simulink model "reverbatinDelay"  (Simulink 7.7)
settings: Solver=FixedStepDiscrete  StartTime=0.0  StopTime=10.0  RelTol=1e-3
libraries: dspsigops x1, dspsrcs4 x1, dspmtrx3 x1, dspsnks4 x1
settings Model: Creator=Arun  LastModifiedBy=Arun

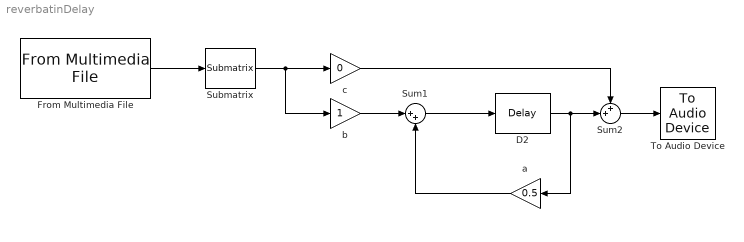
== system reverbatinDelay ==
  D2 : dspsigops/Delay  InputProcessing=Columns as channels (frame based)  dly_unit=Samples  delay=6000  ic_detail=off  dif_ic_for_ch=off  dif_ic_for_dly=off  ic=0  reset_popup=None
  From Multimedia File : dspsrcs4/From Multimedia File  inputFilename=I:\Documents and Settings\Arun\Desktop\monayi\speech_dft.wav  loop=on  numPlays=1  outputStreams=Audio only  videoDataType=single  audioDataType=double  inheritSampleTime=on  userDefinedSampleTime=1/30  noAudioOutput=off  isIntensityVideo=off  fourcc=RGB  colorVideoFormat=Separate color signals  outputEOF=off  dataOrg=Column-major  audioFrameSize=1  computeAudioFrameSize=off
  Submatrix : dspmtrx3/Submatrix  RowSpan=All rows  RowStartMode=First  RowStartIndex=1  RowEndMode=Last  RowEndIndex=1  ColSpan=One column  ColStartMode=First  ColStartIndex=1  ColEndMode=Last  ColEndIndex=1
  Sum1 : Sum  Inputs=|++
  Sum2 : Sum  Inputs=++|
  To Audio Device : dspsnks4/To Audio Device  deviceName=Default  inheritSampleRate=on  sampleRate=44100  deviceDatatype=Determine from input data type  autoBufferSize=on  bufferSize=4096  queueDuration=1.0
  a : Gain  Gain=0.5
  b : Gain
  c : Gain  Gain=0
  wires:
  From Multimedia File/1 -> Submatrix/1
  Submatrix/1 -> c/1, b/1
  c/1 -> Sum2/1
  D2/1 -> Sum2/2, a/1
  b/1 -> Sum1/1
  Sum1/1 -> D2/1
  a/1 -> Sum1/2
  Sum2/1 -> To Audio Device/1
